simulink model "Rasp"  (R2024a)
settings: Solver=FixedStepAuto  StartTime=0.0  StopTime=20  FixedStep=Ts  RelTol=1e-3  EnableMultiTasking=on
values from neighbouring files (symbols this model uses):
  Ac = [1 0 0 0 0 0 0 0;       -1 0 0 0 0 0 0 0;       0 1 0 0 0 0 0 0;       0 -1 0 0 0 0 0 0;       0 0 1 0 0 0 0 0;       0 0 -1 0 0 0 0 0;       0 0 0 1 0 0 0 0;       0 0 0 -1 0 0 0 0;       0 0 0 0 1 0 0 0;       0 0 0 0 -1 0 0 0;       0 0 0 0 0 1 0 0;       0 0 0 0 0 -1 0 0;       0 0 0 0 0 0 1 0;       0 0 0 0 0 0 -1 0;       0 0 0 0 0 0 0 1;       0 0 0 0 0 0 0 -1;        ]    [load_example_QProblem.m]
  b0 = 12*ones(2*N,1)    [load_example_QProblem.m]
  C = sysd.C    [load_example_QProblem.m]    (also in lqrandmpc.m = linsys1_C.C)
  F = F_bar'    [load_example_QProblem.m]
  H = Linv    [load_example_QProblem.m]
  k_lqr = H\F_bar'    [load_example_QProblem.m]
  N = 8    [load_example_QProblem.m]
  Ts = 0.01    [load_example_QProblem.m]    (also in lqrandmpc.m)
undefined symbols (not defined in the file or in its folder): KA_D, KA_P, rad, s, sigbuilder_block
libraries: raspberrypiBasiclib x14, simulink x14, raspberrypiCommlib x3, aerolibconvert2 x2, simulink_extras x2, eeGeneralControl x2, mpclib x2, slctrl_fre x1, slpidlib x1, eeStairGenerator x1
settings Model: ExtModeTrigDuration=2  Creator=Muham  LastModifiedBy=muham
settings SolverCC: PositivePriorityOrder=on  AutoInsertRateTranBlk=on
settings DataIOCC: SaveFormat=StructureWithTime  SaveOutput=off  SaveTime=off
settings OptimizationCC: ReuseModelBlockBuffer=off  EnhancedBackFolding=on  PassReuseOutputArgsAs=Individual arguments  ZeroExternalMemoryAtStartup=off  ZeroInternalMemoryAtStartup=off  MaxStackSize=64  OptimizeBlockOrder=speed  DifferentSizesBufferReuse=on  EfficientTunableParamExpr=on
settings DebuggingCC: ParameterTunabilityLossMsg=error  UnconnectedInputMsg=warning  UnconnectedOutputMsg=warning  UnconnectedLineMsg=warning
settings HardwareCC: ProdBitPerPointer=32  ProdBitPerSizeT=32  ProdBitPerPtrDiffT=32  ProdLargestAtomicInteger=Long  ProdLargestAtomicFloat=Double  ProdWordSize=32  ProdLongLongMode=on  ProdHWDeviceType=ARM Compatible->ARM Cortex
settings ModelReferenceCC: EnableRefExpFcnMdlSchedulingChecks=on
settings RTWCC: Description=Embedded Coder  SystemTargetFile=ert.tlc  HardwareBoard=Raspberry Pi  TLCOptions="-aInlineSetEventsForThisBaseRateFcn=TLC_FALSE -aSuppressMultiTaskScheduler=TLC_FALSE  -aRateBasedStepFcn=0"  TemplateMakefile=ert_default_tmf  Toolchain=GNU GCC Embedded Linux  BuildConfiguration=Faster Runs  GPUComputeCapability=3.5  DLArmComputeVersion=19.05
settings CodeAppCC: ForceParamTrailComments=on  IgnoreCustomStorageClasses=off  OperatorAnnotations=on  SimulinkDataObjDesc=on  SFDataObjDesc=on  InsertBlockDesc=on
settings ERTTargetCC: SupportContinuousTime=on  SupportVariableSizeSignals=on  ExtModeTransport=2  ExtModeStaticAlloc=on  ExtModeMexFile=ext_xcp  ExtModeIntrfLevel=Level2 - Open

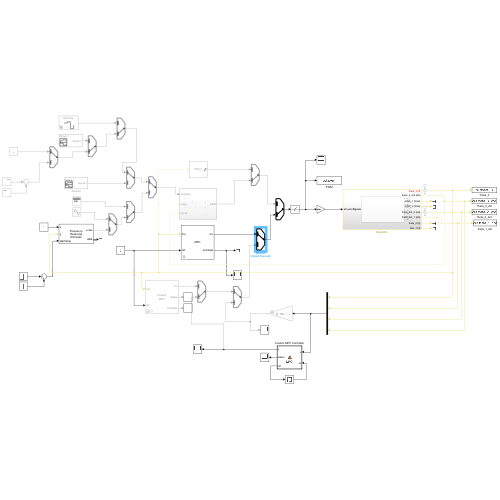
[thumbnail: Simulink's stored preview of the top-level diagram]
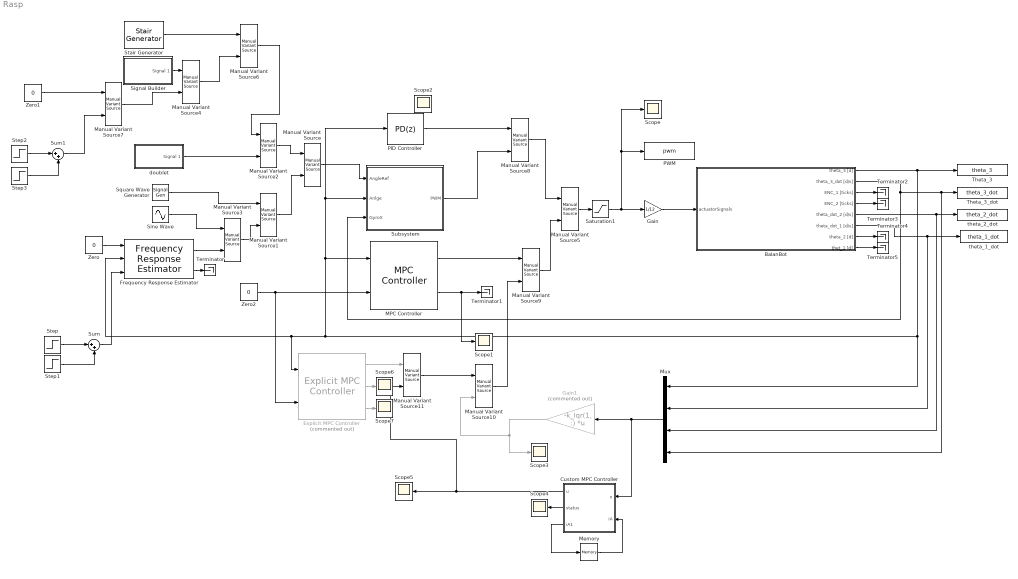
== system Rasp ==
  BalanBot : Subsystem
  Custom MPC Controller : MATLAB Function  TreatAsAtomicUnit=on
  Explicit MPC Controller : mpclib/Explicit MPC Controller  Commented=on  SCDEnableBlockLinearizationSpecification=on  empcobj=empcobj  is_multiple=0  enable_value=0  return_u0=off  md_inport=off  mv_inport=off  return_status=on  return_region=off  return_state=on  state_inport=off  BlockDataType=double  SampleTimeInherited=off  switch_inport=off
  Frequency Response Estimator : slctrl_fre/Frequency Response Estimator  DiscreteTs=Ts  OutputMode=control action + perturbation  BlockDataType=double  SineSource=Block parameters  Frequencies=[2 1 1]  FreqUnits=Hz  Amplitudes=[8 5 2]  NumOfFreq=3  ExperimentMode=Sinestream  NumOfSetPeriod=2  NumOfEstPeriod=4  NumOfSlowestPeriod=3  NumOfPRBSPeriod=1  UseAutogenNumOfPRBSPeriod=off  PRBSSignalOrder=10  UseAutogenPRBSSignalOrder=off  EstimationMode=Offline  UseBodePlot=off  BaselinePlant=[]  PlotRefreshFactor=100  UseExternalTs=off  BodePlotChoice=VariantNull  ExperimentChoice=VariantSSNoEst  OutputChoice=VariantCandD  CompiledTsChoice=InternalTs
  Gain : Gain  Gain=1/12
  Gain1 : Gain  Commented=on  Gain=-k_lqr(1, :)  Multiplication=Matrix(K*u)
  MPC Controller : mpclib/MPC Controller  SCDEnableBlockLinearizationSpecification=on  mpcobj=mpc1  is_multiple=0  enable_value=0  return_u0=off  updateMPCinCallerWorkspace=on  md_inport=off  mv_inport=off  uref_inport=off  return_cost=off  return_mvseq=off  return_qpstatus=off  return_xseq=off  return_state=on  return_ovseq=off  state_inport=off  umin_inport=off  umax_inport=off  ymin_inport=off  ymax_inport=off  cc_inport=off  ywt_inport=off  uwt_inport=off  duwt_inport=off  rhoeps_inport=off  pm_inport=off  MaximumP=100  HorizonChoice=FixedHorizon  n_ts=0.01  n_p=40  n_mv=1  n_md=0  n_ud=0  n_mo=1  n_uo=0  BlockDataType=double  SampleTimeInherited=off  switch_inport=off
  Manual Variant Source{,2..3,7,9..10} (6 alike) : simulink/Signal Routing/Manual Variant Source  NumChoices=2  LabelModeActiveChoice=V_1
  Manual Variant Source{1,4..6,8,11} (6 alike) : simulink/Signal Routing/Manual Variant Source  NumChoices=2  LabelModeActiveChoice=V_2
  Memory : Memory  InitialCondition=false(2*N,1)
  Mux : Mux
  PID Controller : slpidlib/PID Controller  Controller=PD  Form=Parallel  TimeDomain=Discrete-time  UseExternalTs=off  SampleTime=Ts  IntegratorMethod=Trapezoidal  FilterMethod=Forward Euler  ControllerParametersSource=internal  P=12  I=C.Ti  UseKiTs=off  D=0.39  UseExternalDerivativeSource=off  N=100  UseFilter=off  TunerSelectOption=Transfer Function Based (PID Tuner App)  InitialConditionSource=internal  InitialConditionForIntegrator=0  InitialConditionForFilter=0  DifferentiatorICPrevScaledInput=0  ExternalReset=none  TrackingMode=off  Kt=1  LimitOutput=on  SatLimitsSource=internal  UpperSaturationLimit=255  LowerSaturationLimit=-255  LinearizeAsGain=on  AntiWindupMode=none  Kb=1  LimitIntegrator=off  UpperIntegratorSaturationLimit=inf  LowerIntegratorSaturationLimit=-inf  POutMin=[]  POutMax=[]  IOutMin=[]  IOutMax=[]  DOutMin=[]  DOutMax=[]  NOutMin=[]  NOutMax=[]  SumOutMin=[]  SumOutMax=[]  SaturationOutMin=[]  SaturationOutMax=[]  PParamMin=[]  PParamMax=[]  IParamMin=[]  IParamMax=[]  DParamMin=[]  DParamMax=[]  NParamMin=[]  NParamMax=[]  KbParamMin=[]  KbParamMax=[]  KtParamMin=[]  KtParamMax=[]  KbOutMin=[]  KbOutMax=[]  KtOutMin=[]  KtOutMax=[]  IntegratorOutMin=[]  IntegratorOutMax=[]  FilterOutMin=[]  FilterOutMax=[]  SumI1OutMin=[]  SumI1OutMax=[]  SumI2OutMin=[]  SumI2OutMax=[]  SumI3OutMin=[]  SumI3OutMax=[]  SumI4OutMin=[]  SumI4OutMax=[]  SumDOutMin=[]  SumDOutMax=[]  DifferentiatorOutMin=[]  DifferentiatorOutMax=[]  FilterDiffOutCoefMin=[]  FilterDiffOutCoefMax=[]  ReciprocalOutMin=[]  ReciprocalOutMax=[]  SumDenOutMin=[]  SumDenOutMax=[]  SumNumOutMin=[]  SumNumOutMax=[]  DivideOutMin=[]  DivideOutMax=[]  UdiffTsProdOutMin=[]  UdiffTsProdOutMax=[]  NTsProdOutMin=[]  NTsProdOutMax=[]  UintegralTsProdOutMin=[]  UintegralTsProdOutMax=[]  UngainTsProdOutMin=[]  UngainTsProdOutMax=[]  ClampingZeroOutDataTypeStr=Inherit: Inherit via back propagation  ClampingZeroOutMin=[]  ClampingZeroOutMax=[]  FilterDenConstantOutDataTypeStr=Inherit: Inherit via back propagation  FilterDenConstantOutMin=[]  FilterDenConstantOutMax=[]  PCopyOutDataTypeStr=Inherit: Inherit via back propagation  PCopyOutMin=[]  PCopyOutMax=[]  NCopyOutDataTypeStr=Inherit: Inherit via back propagation  NCopyOutMin=[]  NCopyOutMax=[]  IntegratorContinuousStateAttributes=''  IntegratorStateMustResolveToSignalObject=off  IntegratorRTWStateStorageClass=Auto  FilterContinuousStateAttributes=''  FilterStateMustResolveToSignalObject=off  FilterRTWStateStorageClass=Auto  ParallelPVariant=InternalParameters  IdealPVariant=Disabled  IVariant=Disabled  DVariant=InternalParameters  IntegratorVariant=Disabled  SatVariant=Enabled  AWVariant=Disabled  PCopyVariant=Disabled  TRVariant=Disabled  FdbkBlocksVariant=Forward  IdealPFdbkVariant=Disabled  SatFdbkVariant=Disabled  DerivativeFilterVariant=Differentiator  NVariant=Passthrough  NCopyVariant=Disabled_SignalSpec  FilterICVariant=InternalICsDifferentiator  IntegratorICVariant=Disabled  ExternalResetVariant=Disabled  TRSumVariant=Passthrough  SumFdbkVariant=Disabled  SumVariant=Sum_PD  TsampFilterVariant=InternalTs  TsampNgainVariant=Passthrough  TsampIntegralVariant=Disabled_SignalSpec  ExternalSaturationOutDataTypeStr=Inherit: Same as second input  DerivativeSourceVariant=ErrorSignal
  PWM : ToWorkspace  VariableName=pwm  SaveFormat=Timeseries  SampleTime=Ts
  Saturation1 : Saturate  UpperLimit=12  LowerLimit=-12
  Scope{,1..7} (8 alike) : Scope
  Signal Builder : Subsystem  Tag=STV Subsys  LoadFcn=sigbuilder_block('load');  StartFcn=sigbuilder_block('start');  StopFcn=sigbuilder_block('stop');  ClipboardFcn=sigbuilder_block('clipboard');  mask(Sigbuilder block){tuvar=[0:10]}
      mask help: Simulink:masks:SigbuilderBlock_MD
      mask init:
      | if ~strcmp(get_param(bdroot(gcbh),'SimulationStatus'),'stopped') tuvar = sigbuilder_block('maskInit'); end
      settings: CopyFcn=sigbuilder_block('copy');  DeleteFcn=sigbuilder_block('delete');  ModelCloseFcn=sigbuilder_block('modelClose');  PreSaveFcn=sigbuilder_block('preSave');  PauseFcn=sigbuilder_block('pause');  ContinueFcn=sigbuilder_block('continue');  NameChangeFcn=sigbuilder_block('namechange');  OpenFcn=sigbuilder_block('open',[6 36 1428 675.75 ]);  CloseFcn=sigbuilder_block('close');
      mask Display: plot(0, 0, 100, 100,[2, 2, 32, 32, 2], [68, 8, 8, 68, 68],[32, 2], [38, 38], [32, 19, 2],[53, 60, 44], [32, 17, 17, 2],[16, 16, 31, 31]);txt = getActiveGroup(gcbh);text(2, 100, txt,'verticalAlignment', 'top');
  Sine Wave : Sin  Amplitude=5  Frequency=6.2831853  SampleTime=Ts
  Square Wave Generator : SignalGenerator  WaveForm=square  Amplitude=8
  Stair Generator : eeStairGenerator/Stair Generator  LabelModeActiveChoice=Discrete  TimeInput=[5 10 15 20]  AmplitudeInput=[5 8 -8 0]  SampleTime=-1  RepeatPattern=on  OutDataTypeStr=double
      settings: LibrarySourceBlock=ee_sl_lib/General Control/Stair Generator
  Step : Step  Time=5  SampleTime=Ts
  Step1 : Step  Time=21  After=-1  SampleTime=Ts
  Step2 : Step  Time=5  After=5  SampleTime=0
  Step3 : Step  Time=5.1  After=-5  SampleTime=0
  Subsystem : Subsystem
  Sum : Sum  Inputs=|++
  Sum1 : Sum  Inputs=|++
  Terminator{,1..5} (6 alike) : Terminator
  Theta_3 : ToWorkspace  VariableName=theta_3  SaveFormat=Timeseries  SampleTime=Ts
  Theta_3_dot : ToWorkspace  VariableName=theta_3_dot  SaveFormat=Timeseries  SampleTime=Ts
  Zero : Constant  Value=0  OutDataTypeStr=Inherit: Inherit via back propagation
  Zero1 : Constant  Value=0  OutDataTypeStr=Inherit: Inherit via back propagation  SampleTime=Ts
  Zero2 : Constant  Value=0  OutDataTypeStr=Inherit: Inherit via back propagation
  doublet : Subsystem  Tag=STV Subsys  LoadFcn=sigbuilder_block('load');  StartFcn=sigbuilder_block('start');  StopFcn=sigbuilder_block('stop');  ClipboardFcn=sigbuilder_block('clipboard');  mask(Sigbuilder block){tuvar=[0:10]}
      mask help: Simulink:masks:SigbuilderBlock_MD
      mask init:
      | if ~strcmp(get_param(bdroot(gcbh),'SimulationStatus'),'stopped') tuvar = sigbuilder_block('maskInit'); end
      settings: CopyFcn=sigbuilder_block('copy');  DeleteFcn=sigbuilder_block('delete');  ModelCloseFcn=sigbuilder_block('modelClose');  PreSaveFcn=sigbuilder_block('preSave');  PauseFcn=sigbuilder_block('pause');  ContinueFcn=sigbuilder_block('continue');  NameChangeFcn=sigbuilder_block('namechange');  OpenFcn=sigbuilder_block('open',[6 0 1428 711.75 ]);  CloseFcn=sigbuilder_block('close');
      mask Display: plot(0, 0, 100, 100,[2, 2, 32, 32, 2], [68, 8, 8, 68, 68],[32, 2], [38, 38], [32, 19, 2],[53, 60, 44], [32, 17, 17, 2],[16, 16, 31, 31]);txt = getActiveGroup(gcbh);text(2, 100, txt,'verticalAlignment', 'top');
  theta_1_dot : ToWorkspace  VariableName=theta_1_dot  SaveFormat=Timeseries  SampleTime=Ts
  theta_2_dot : ToWorkspace  VariableName=theta_2_dot  SaveFormat=Timeseries  SampleTime=Ts
  wires:
  BalanBot/2(theta_3_dot [d/s]) -> Subsystem/3(GyroX), Mux/4, Theta_3_dot/1
  Manual Variant Source1/1 -> Manual Variant Source/2
  Square Wave Generator/1 -> Manual Variant Source1/1
  Manual Variant Source2/1 -> Manual Variant Source/1
  doublet/1(Signal 1) -> Manual Variant Source2/2
  Manual Variant Source3/1 -> Manual Variant Source1/2
  Sine Wave/1 -> Manual Variant Source3/1
  Frequency Response Estimator/1 -> Manual Variant Source3/2
  Step1/1 -> Sum/2
  Sum/1 -> Frequency Response Estimator/3
  Step/1 -> Sum/1
  Zero/1 -> Frequency Response Estimator/1
  Frequency Response Estimator/2 -> Terminator/1
  Signal Builder/1(Signal 1) -> Manual Variant Source4/1
  Stair Generator/1 -> Manual Variant Source6/1
  Manual Variant Source6/1 -> Manual Variant Source2/1
  Manual Variant Source4/1 -> Manual Variant Source6/2
  Zero1/1 -> Manual Variant Source7/1
  Manual Variant Source7/1 -> Manual Variant Source4/2
  Step2/1 -> Sum1/1
  Step3/1 -> Sum1/2
  Sum1/1 -> Manual Variant Source7/2
  Manual Variant Source5/1 -> Saturation1/1
  Gain/1 -> BalanBot/1(actuatorSignals)
  Saturation1/1 -> Scope/1, PWM/1, Gain/1
  MPC Controller/2 -> Scope1/1, Terminator1/1
  BalanBot/1(theta_3 [d]) -> Theta_3/1, Mux/1, Explicit MPC Controller/1, Frequency Response Estimator/2, PID Controller/1, Subsystem/2(Anlge), MPC Controller/1
  BalanBot/3(ENC_1 [ticks]) -> Terminator2/1
  BalanBot/4(ENC_2 [ticks]) -> Terminator3/1
  BalanBot/5(theta_dot_2 [d/s]) -> theta_2_dot/1, Mux/3
  BalanBot/6(theta_dot_1 [d/s]) -> theta_1_dot/1, Mux/2
  BalanBot/7(theta_2 [d]) -> Terminator4/1
  BalanBot/8(thet_1 [d]) -> Terminator5/1
  Subsystem/1(PWM) -> Manual Variant Source8/2
  Manual Variant Source8/1 -> Manual Variant Source5/1
  PID Controller/1 -> Manual Variant Source8/1
  Manual Variant Source9/1 -> Manual Variant Source5/2
  MPC Controller/1 -> Manual Variant Source9/1
  Gain1/1 -> Manual Variant Source10/2, Scope3/1
  Manual Variant Source/1 -> Subsystem/1(AngleRef)
  Mux/1 -> Custom MPC Controller/1(x), Gain1/1
  Custom MPC Controller/3(iA1) -> Memory/1
  Memory/1 -> Custom MPC Controller/2(iA)
  Manual Variant Source10/1 -> Manual Variant Source9/2
  Custom MPC Controller/2(status) -> Scope4/1
  Custom MPC Controller/1(u) -> Manual Variant Source11/2, Scope5/1
  Zero2/1 -> Explicit MPC Controller/2, MPC Controller/2
  Explicit MPC Controller/1 -> Manual Variant Source11/1
  Manual Variant Source11/1 -> Manual Variant Source10/1
  Explicit MPC Controller/2 -> Scope6/1
  Explicit MPC Controller/3 -> Scope7/1

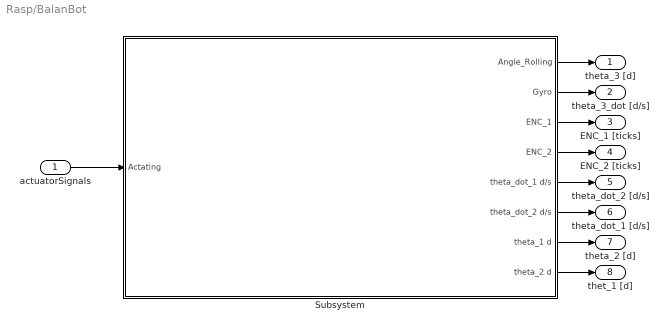
== system Rasp/BalanBot ==
  actuatorSignals : Inport
  Subsystem : Subsystem  VariantControl=plantModel==2
  theta_3 [d] : Outport
  theta_3_dot [d/s] : Outport  Port=2
  ENC_1 [ticks] : Outport  Port=3
  ENC_2 [ticks] : Outport  Port=4
  theta_dot_2 [d/s] : Outport  Port=5
  theta_dot_1 [d/s] : Outport  Port=6
  theta_2 [d] : Outport  Port=7
  thet_1 [d] : Outport  Port=8
  wires:
  actuatorSignals/1 -> Subsystem/1(Actating)
  Subsystem/1(Angle_Rolling) -> theta_3 [d]/1
  Subsystem/2(Gyro) -> theta_3_dot [d/s]/1
  Subsystem/3(ENC_1) -> ENC_1 [ticks]/1
  Subsystem/4(ENC_2) -> ENC_2 [ticks]/1
  Subsystem/5(theta_dot_1 d/s) -> theta_dot_2 [d/s]/1
  Subsystem/6(theta_dot_2 d/s) -> theta_dot_1 [d/s]/1
  Subsystem/7(theta_1 d) -> theta_2 [d]/1
  Subsystem/8(theta_2 d) -> thet_1 [d]/1

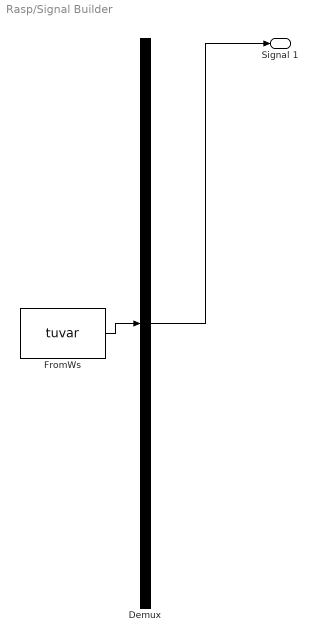
== system Rasp/Signal Builder ==
  Demux : Demux  Tag=STV Demux  Outputs=1
      settings: DisplayOption=none
  FromWs : FromWorkspace  Tag=STV FromWs  VariableName=tuvar
      SigBuilderData=|
      | common.afterFinalStr = 'Extrapolate'
      | common.sampleTime = 0
      | dataSet.timeRange = [0 6]
      | dataSet.name = 'Group 1'
      | sbobj.Groups.Name = 'Group 1'
      | sbobj.Groups.Signals.Name = 'Signal 1'
      | sbobj.Groups.Signals.XData = [0 0.175 0.175 0.205 0.205 3 3 3.1 3.1 4 4 4.1 4.1 5 5 5.1 5.1 6]
      | sbobj.Groups.Signals.YData = [0 0 5 5 0.002 0 10 10 0 0.00260869565217 -10 -10 0.00388405797101 0 -5 -5 0 0.00367346938776]
      | sbobj.Groups.TimeRange = [0 6]
  Signal 1 : Outport  Tag=STV Outport
  wires:
  Demux/1 -> Signal 1/1
  FromWs/1 -> Demux/1

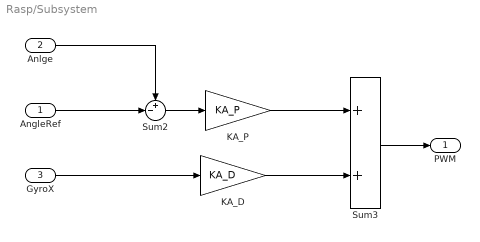
== system Rasp/Subsystem ==
  AngleRef : Inport
  Anlge : Inport  Port=2
  GyroX : Inport  Port=3
  KA_D : Gain  Gain=KA_D
  KA_P : Gain  Gain=KA_P
  Sum2 : Sum  Inputs=+-|
  Sum3 : Sum
  PWM : Outport
  wires:
  GyroX/1 -> KA_D/1
  KA_P/1 -> Sum3/1
  Sum2/1 -> KA_P/1
  KA_D/1 -> Sum3/2
  Anlge/1 -> Sum2/1
  AngleRef/1 -> Sum2/2
  Sum3/1 -> PWM/1

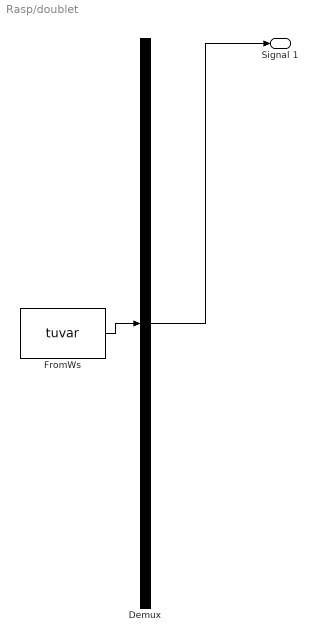
== system Rasp/doublet ==
  Demux : Demux  Tag=STV Demux  Outputs=1
      settings: DisplayOption=none
  FromWs : FromWorkspace  Tag=STV FromWs  VariableName=tuvar
      SigBuilderData=|
      | common.afterFinalStr = 'Extrapolate'
      | common.sampleTime = 0
      | dataSet.timeRange = [0 15]
      | dataSet.name = 'Group 1'
      | sbobj.Groups.Name = 'Group 1'
      | sbobj.Groups.Signals.Name = 'Signal 1'
      | sbobj.Groups.Signals.XData = [0 2.61 2.61 2.64 2.64 8.44 8.44 8.46 8.46 13.58 13.58 13.61 13.61 15]
      | sbobj.Groups.Signals.YData = [0 0 -5 -5 -0.02 0 4.92 4.92 0 0 -4.36 -4.36 0 0]
      | sbobj.Groups.TimeRange = [0 15]
  Signal 1 : Outport  Tag=STV Outport
  wires:
  Demux/1 -> Signal 1/1
  FromWs/1 -> Demux/1

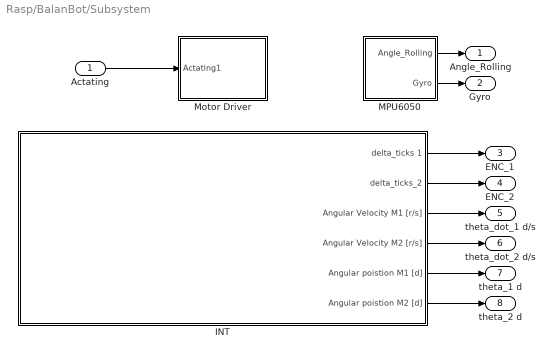
== system Rasp/BalanBot/Subsystem ==
  Actating : Inport
  INT : Subsystem
  MPU6050 : Subsystem
  Motor Driver : Subsystem
  Angle_Rolling : Outport
  Gyro : Outport  Port=2
  ENC_1 : Outport  Port=3
  ENC_2 : Outport  Port=4
  theta_dot_1 d/s : Outport  Port=5
  theta_dot_2 d/s : Outport  Port=6
  theta_1 d : Outport  Port=7
  theta_2 d : Outport  Port=8
  wires:
  Actating/1 -> Motor Driver/1(Actating1)
  INT/1(delta_ticks 1) -> ENC_1/1
  INT/2(delta_ticks_2) -> ENC_2/1
  INT/3(Angular Velocity M1 [r/s]) -> theta_dot_1 d/s/1
  INT/4(Angular Velocity M2 [r/s]) -> theta_dot_2 d/s/1
  INT/5(Angular poistion M1 [d]) -> theta_1 d/1
  INT/6(Angular poistion M2 [d]) -> theta_2 d/1
  MPU6050/2(Gyro) -> Gyro/1
  MPU6050/1(Angle_Rolling) -> Angle_Rolling/1

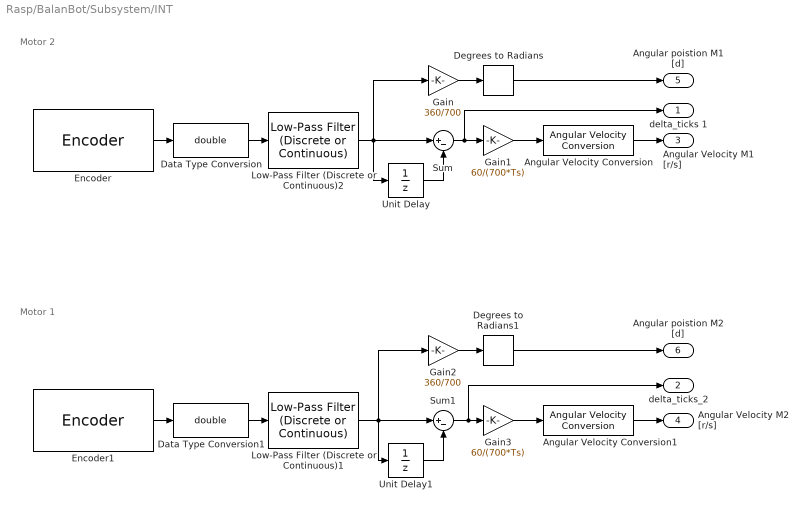
== system Rasp/BalanBot/Subsystem/INT ==
  note: Motor 2
  note: Motor 1
  Angular Velocity Conversion : aerolibconvert2/Angular Velocity Conversion  IU=rpm  OU=rad/s
  Angular Velocity Conversion1 : aerolibconvert2/Angular Velocity Conversion  IU=rpm  OU=rad/s
  Data Type Conversion : DataTypeConversion  OutDataTypeStr=double  SaturateOnIntegerOverflow=off  RndMeth=Floor
  Data Type Conversion1 : DataTypeConversion  OutDataTypeStr=double  SaturateOnIntegerOverflow=off  RndMeth=Floor
  Degrees to Radians : simulink_extras/Transformations/Degrees to Radians
  Degrees to Radians1 : simulink_extras/Transformations/Degrees to Radians
  Encoder : raspberrypiBasiclib/Encoder  BoardProperty=Pi 4 Model B  InputA=GPIO 20  InputB=GPIO 21  Mode=No reset  SampleTime=-1
  Encoder1 : raspberrypiBasiclib/Encoder  BoardProperty=Pi 4 Model B  InputA=GPIO 26  InputB=GPIO 19  Mode=No reset  SampleTime=-1
  Gain : Gain  Gain=360/700
  Gain1 : Gain  Gain=60/(700*Ts)
  Gain2 : Gain  Gain=360/700
  Gain3 : Gain  Gain=60/(700*Ts)
  Low-Pass Filter (Discrete or Continuous)1 : eeGeneralControl/Low-Pass Filter (Discrete or Continuous)  K=1  T=Ts * 10  B=inf  A=-inf  init_option=Inherited from block input  x0=0  Ts=-1
  Low-Pass Filter (Discrete or Continuous)2 : eeGeneralControl/Low-Pass Filter (Discrete or Continuous)  K=1  T=Ts * 10  B=inf  A=-inf  init_option=Inherited from block input  x0=0  Ts=-1
  Sum : Sum  Inputs=|+-
  Sum1 : Sum  Inputs=|+-
  Unit Delay : UnitDelay  SampleTime=-1  HasFrameUpgradeWarning=on
  Unit Delay1 : UnitDelay  SampleTime=-1  HasFrameUpgradeWarning=on
  delta_ticks 1 : Outport
  delta_ticks_2 : Outport  Port=2
  Angular Velocity M1 [r/s] : Outport  Port=3
  Angular Velocity M2 [r/s] : Outport  Port=4
  Angular poistion M1 [d] : Outport  Port=5
  Angular poistion M2 [d] : Outport  Port=6
  wires:
  Encoder/1 -> Data Type Conversion/1
  Encoder1/1 -> Data Type Conversion1/1
  Data Type Conversion/1 -> Low-Pass Filter (Discrete or Continuous)2/1
  Sum/1 -> delta_ticks 1/1, Gain1/1
  Sum1/1 -> delta_ticks_2/1, Gain3/1
  Data Type Conversion1/1 -> Low-Pass Filter (Discrete or Continuous)1/1
  Low-Pass Filter (Discrete or Continuous)2/1 -> Gain/1, Sum/1, Unit Delay/1
  Unit Delay/1 -> Sum/2
  Gain1/1 -> Angular Velocity Conversion/1
  Angular Velocity Conversion/1 -> Angular Velocity M1 [r/s]/1
  Gain/1 -> Degrees to Radians/1
  Degrees to Radians/1 -> Angular poistion M1 [d]/1
  Angular Velocity Conversion1/1 -> Angular Velocity M2 [r/s]/1
  Gain3/1 -> Angular Velocity Conversion1/1
  Gain2/1 -> Degrees to Radians1/1
  Unit Delay1/1 -> Sum1/2
  Low-Pass Filter (Discrete or Continuous)1/1 -> Gain2/1, Sum1/1, Unit Delay1/1
  Degrees to Radians1/1 -> Angular poistion M2 [d]/1

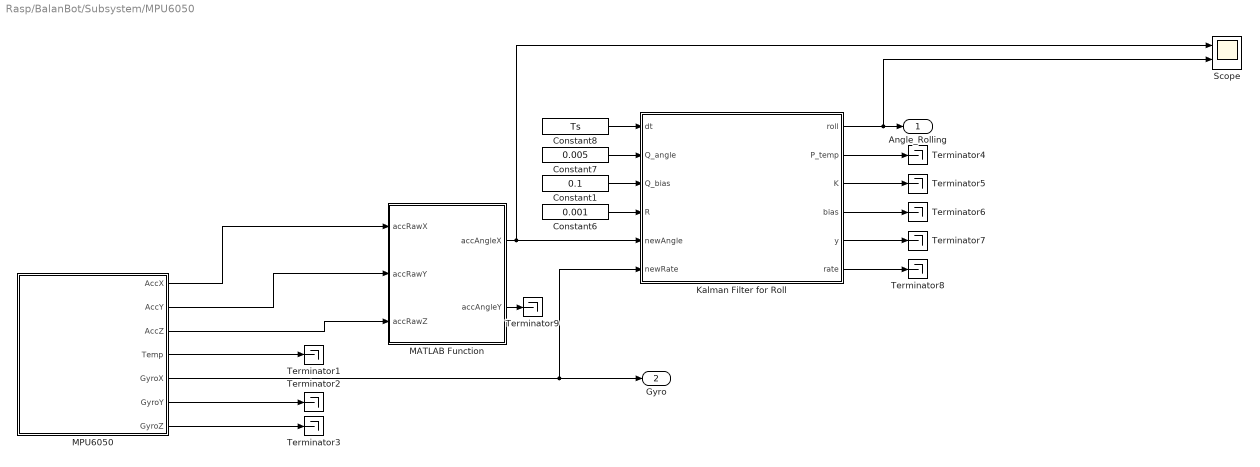
== system Rasp/BalanBot/Subsystem/MPU6050 ==
  Constant1 : Constant  Value=0.1
  Constant6 : Constant  Value=0.001
  Constant7 : Constant  Value=0.005
  Constant8 : Constant  Value=Ts
  Kalman Filter for Roll : MATLAB Function  TreatAsAtomicUnit=on
  MATLAB Function : MATLAB Function  TreatAsAtomicUnit=on
  MPU6050 : Subsystem  TreatAsAtomicUnit=on
  Scope : Scope  NumInputPorts=2
  Terminator{1..9} (9 alike) : Terminator
  Angle_Rolling : Outport
  Gyro : Outport  Port=2
  wires:
  MPU6050/7(GyroZ) -> Terminator3/1
  MPU6050/5(GyroX) -> Kalman Filter for Roll/6(newRate), Gyro/1
  MPU6050/2(AccY) -> MATLAB Function/2(accRawY)
  MPU6050/3(AccZ) -> MATLAB Function/3(accRawZ)
  MPU6050/4(Temp) -> Terminator1/1
  MPU6050/1(AccX) -> MATLAB Function/1(accRawX)
  Constant8/1 -> Kalman Filter for Roll/1(dt)
  Constant7/1 -> Kalman Filter for Roll/2(Q_angle)
  Constant1/1 -> Kalman Filter for Roll/3(Q_bias)
  Constant6/1 -> Kalman Filter for Roll/4(R)
  Kalman Filter for Roll/1(roll) -> Scope/2, Angle_Rolling/1
  Kalman Filter for Roll/2(P_temp) -> Terminator4/1
  Kalman Filter for Roll/3(K) -> Terminator5/1
  Kalman Filter for Roll/4(bias) -> Terminator6/1
  Kalman Filter for Roll/5(y) -> Terminator7/1
  Kalman Filter for Roll/6(rate) -> Terminator8/1
  MATLAB Function/1(accAngleX) -> Scope/1, Kalman Filter for Roll/5(newAngle)
  MPU6050/6(GyroY) -> Terminator2/1
  MATLAB Function/2(accAngleY) -> Terminator9/1

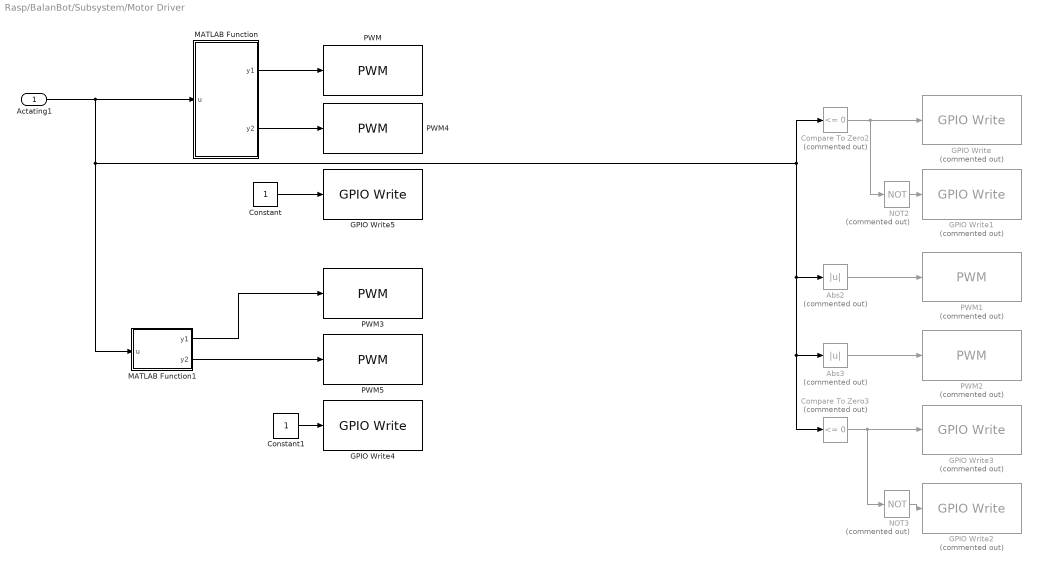
== system Rasp/BalanBot/Subsystem/Motor Driver ==
  Actating1 : Inport
  Abs2 : Abs  Commented=on  SaturateOnIntegerOverflow=off
  Abs3 : Abs  Commented=on  SaturateOnIntegerOverflow=off
  Compare To Zero2 : simulink/Logic and Bit Operations/Compare To Zero  Commented=on  relop=<=  OutDataTypeStr=boolean
  Compare To Zero3 : simulink/Logic and Bit Operations/Compare To Zero  Commented=on  relop=<=  OutDataTypeStr=boolean
  Constant : Constant
  Constant1 : Constant
  GPIO Write : raspberrypiBasiclib/GPIO Write  Commented=on  board=Pi 4 Model B  gpio=27  direction=Output  blockPlatform=Raspberry Pi
  GPIO Write1 : raspberrypiBasiclib/GPIO Write  Commented=on  board=Pi 4 Model B  gpio=22  direction=Output  blockPlatform=Raspberry Pi
  GPIO Write2 : raspberrypiBasiclib/GPIO Write  Commented=on  board=Pi 4 Model B  gpio=15  direction=Output  blockPlatform=Raspberry Pi
  GPIO Write3 : raspberrypiBasiclib/GPIO Write  Commented=on  board=Pi 4 Model B  gpio=18  direction=Output  blockPlatform=Raspberry Pi
  GPIO Write4 : raspberrypiBasiclib/GPIO Write  board=Pi 4 Model B  gpio=14  direction=Output  blockPlatform=Raspberry Pi
  GPIO Write5 : raspberrypiBasiclib/GPIO Write  board=Pi 4 Model B  gpio=17  direction=Output  blockPlatform=Raspberry Pi
  MATLAB Function : MATLAB Function  TreatAsAtomicUnit=on
  MATLAB Function1 : MATLAB Function  TreatAsAtomicUnit=on
  NOT2 : Logic  Commented=on  Operator=NOT  IconShape=distinctive  AllPortsSameDT=off  OutDataTypeStr=boolean
  NOT3 : Logic  Commented=on  Operator=NOT  IconShape=distinctive  AllPortsSameDT=off  OutDataTypeStr=boolean
  PWM : raspberrypiBasiclib/PWM  board=Pi 2 Model B  Pin_=27  Frequency=8000  blockPlatform=Raspberry Pi
  PWM1 : raspberrypiBasiclib/PWM  Commented=on  board=Pi 4 Model B  Pin_=17  Frequency=1000  blockPlatform=Raspberry Pi
  PWM2 : raspberrypiBasiclib/PWM  Commented=on  board=Pi 4 Model B  Pin_=14  Frequency=1000  blockPlatform=Raspberry Pi
  PWM3 : raspberrypiBasiclib/PWM  board=Pi 2 Model B  Pin_=18  Frequency=8000  blockPlatform=Raspberry Pi
  PWM4 : raspberrypiBasiclib/PWM  board=Pi 2 Model B  Pin_=22  Frequency=8000  blockPlatform=Raspberry Pi
  PWM5 : raspberrypiBasiclib/PWM  board=Pi 2 Model B  Pin_=15  Frequency=8000  blockPlatform=Raspberry Pi
  wires:
  Compare To Zero2/1 -> GPIO Write/1, NOT2/1
  Abs3/1 -> PWM2/1
  NOT3/1 -> GPIO Write2/1
  Compare To Zero3/1 -> GPIO Write3/1, NOT3/1
  NOT2/1 -> GPIO Write1/1
  Abs2/1 -> PWM1/1
  Actating1/1 -> MATLAB Function/1(u), Abs2/1, Compare To Zero3/1, Abs3/1, Compare To Zero2/1, MATLAB Function1/1(u)
  Constant/1 -> GPIO Write5/1
  Constant1/1 -> GPIO Write4/1
  MATLAB Function/2(y2) -> PWM4/1
  MATLAB Function/1(y1) -> PWM/1
  MATLAB Function1/2(y2) -> PWM5/1
  MATLAB Function1/1(y1) -> PWM3/1

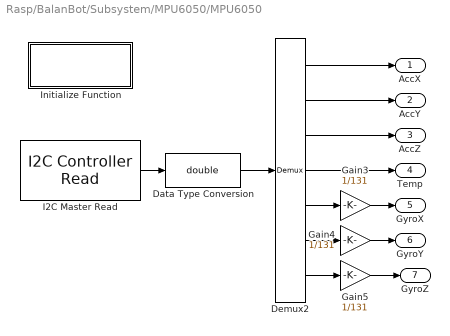
== system Rasp/BalanBot/Subsystem/MPU6050/MPU6050 ==
  Data Type Conversion : DataTypeConversion  OutDataTypeStr=double  SaturateOnIntegerOverflow=off  RndMeth=Floor
  Demux2 : Demux  Outputs=7
  Gain3 : Gain  Gain=1/131
  Gain4 : Gain  Gain=1/131
  Gain5 : Gain  Gain=1/131
  I2C Master Read : raspberrypiCommlib/I2C Controller Read  BoardProperty=Pi 4 Model B  I2CModule=1  Mode=Master  SlaveAddress=hex2dec('68')  SlaveByteOrder=BigEndian  Direction=Receiver  RegisterAddressMode=on  RegisterAddress=hex2dec('3B')  SlaveDataType=int16  DataLength=7  NoAck=off  RepeatedStart=off  OutputStatus=off  SampleTime=-1
  Initialize Function : Subsystem  TreatAsAtomicUnit=on
  AccX : Outport
  AccY : Outport  Port=2
  AccZ : Outport  Port=3
  Temp : Outport  Port=4
  GyroX : Outport  Port=5
  GyroY : Outport  Port=6
  GyroZ : Outport  Port=7
  wires:
  Data Type Conversion/1 -> Demux2/1
  Demux2/5 -> Gain3/1
  I2C Master Read/1 -> Data Type Conversion/1
  Demux2/4 -> Temp/1
  Demux2/6 -> Gain4/1
  Demux2/7 -> Gain5/1
  Demux2/1 -> AccX/1
  Demux2/2 -> AccY/1
  Demux2/3 -> AccZ/1
  Gain3/1 -> GyroX/1
  Gain4/1 -> GyroY/1
  Gain5/1 -> GyroZ/1

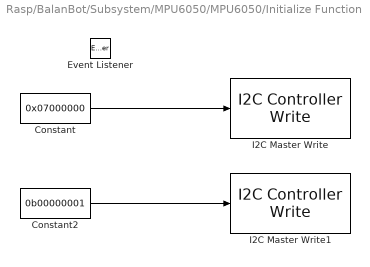
== system Rasp/BalanBot/Subsystem/MPU6050/MPU6050/Initialize Function ==
  Constant : Constant  Value=0x07000000  SampleTime=-1
  Constant2 : Constant  Value=0b00000001  SampleTime=-1
  Event Listener : EventListener  DisableCoverage=on  EventName=reset
  I2C Master Write : raspberrypiCommlib/I2C Controller Write  BoardProperty=Pi 4 Model B  I2CModule=1  Mode=Master  SlaveAddress=uint8(hex2dec('68'))  SlaveByteOrder=BigEndian  Direction=Transmitter  RegisterAddressMode=on  RegisterAddress=uint8(hex2dec('19'))  SlaveDataType=uint8  DataLength=1  NoAck=off  RepeatedStart=off  OutputStatus=off
  I2C Master Write1 : raspberrypiCommlib/I2C Controller Write  BoardProperty=Pi 4 Model B  I2CModule=1  Mode=Master  SlaveAddress=hex2dec('68')  SlaveByteOrder=BigEndian  Direction=Transmitter  RegisterAddressMode=on  RegisterAddress=hex2dec('6B')  SlaveDataType=uint8  DataLength=1  NoAck=off  RepeatedStart=off  OutputStatus=off
  wires:
  Constant2/1 -> I2C Master Write1/1
  Constant/1 -> I2C Master Write/1

== matlab function Rasp/Custom MPC Controller ==
  settings: updateMethod=DISCRETE  sampleTime=Ts
  data: u output; status output; x input; iA input boolean; iA1 output; H parameter; F parameter; Ac parameter; b0 parameter
function [u,status,iA1] = MPC(x,iA,H,F,Ac,b0)
%#codegen
[uMPC,status,iA1] = mpcActiveSetSolver(H,F*x,Ac,b0,[],zeros(0,1),iA,mpcActiveSetOptions("UseHessianAsInput",0,"IntegrityChecks",0));
u = uMPC(1);

== matlab function Rasp/BalanBot/Subsystem/Motor Driver/MATLAB Function ==
  data: u input; y1 output; y2 output
function [y1,y2]= toPWM(u)
if(u <= 0)
    y1 = abs(u);
    y2 = 0;
else
    y1 = 0;
    y2 = abs(u);
end

== matlab function Rasp/BalanBot/Subsystem/Motor Driver/MATLAB Function1 ==
  data: u input; y1 output; y2 output
function [y1,y2]= toPWM(u)
if(u <= 0)
    y1 = abs(u);
    y2 = 0;
else
    y1 = 0;
    y2 = abs(u);
end

== matlab function Rasp/BalanBot/Subsystem/MPU6050/MATLAB Function ==
  data: accRawX input; accAngleX output; accAngleY output; accRawY input; accRawZ input
function [accAngleX, accAngleY] = fcn(accRawX, accRawY, accRawZ)

%Converting the raw accel data from g values to accel about X and Y axis

accAngleX = atand(accRawY/sqrt(power(accRawX,2) + power(accRawZ,2)));
accAngleY = atand(-1*(accRawX/sqrt(power(accRawY,2) + power(accRawZ,2))));

end

== matlab function Rasp/BalanBot/Subsystem/MPU6050/Kalman Filter for Roll ==
  data: dt input; roll output; Q_angle input; Q_bias input; R input; newAngle input; newRate input; P_temp output; K output; bias output; y output; rate output
function [roll, P_temp, K, bias, y, rate]  = kalFilterRoll(dt, Q_angle, Q_bias, R, newAngle, newRate)

persistent angle;
persistent P;


%Process Noise Convariance Matrix
Q = [Q_angle 0; 0 Q_bias] * dt;
F = [1  -dt; 0 1];
H = [1 0];
bias = 0.0;

rate = newRate - bias;

if isempty(angle)
    angle = 0;
else
    angle = angle + (dt * rate);
end 

roll = angle;

if isempty(P)
    P = [0, 0; 0, 0];
else
    P = F*P*F' + Q;
end 
P_temp = P;

S = H*P*H' + R;
K = (P_temp * H')/S;
y = newAngle - roll; 
roll = roll + K(1) * y;
bias = roll + K(2) * y;
angle = roll;

I = [1 0; 0 1];
P_temp = (I - K*H)*P_temp;
P = P_temp;

return 


end
